simulink model "Ball_and_Plate_MicroLabBox_student_v2019"  (R2019b)
settings: Solver=ode1  StartTime=0.0  StopTime=Inf  FixedStep=0.001  RelTol=1e-3
PostLoadFcn:
  | , if any(exist('dsrtsu_mdlpostloadfcn', 'file') ~= 0), dsrtsu_mdlpostloadfcn('Execute', bdroot); end,
InitFcn:
  | , if any(exist('rtifpga_mdlclblib', 'file') ~= 0), rtifpga_mdlclblib('Init', bdroot); end,
values from neighbouring files (symbols this model uses):
  A_robust = K_robust.A    [Init_workspace.m]    (also in OptimalControlleerSythesisNew.m = K.A)
  B_robust = K_robust.B    [Init_workspace.m]    (also in OptimalControlleerSythesisNew.m = K.B)
  ball_pos_sat = 0.2    [Init_workspace.m]
  ball_vel_sat = 1    [Init_workspace.m]
  Baw_robust = C_robust' / (C_robust*C_robust' + aw_reg*eye(2))    [OptimalControlleerSythesisNew.m]
  C_robust = K_robust.C    [Init_workspace.m]    (also in OptimalControlleerSythesisNew.m = K.C)
  D_robust = K_robust.D    [Init_workspace.m]    (also in OptimalControlleerSythesisNew.m = K.D)
  g = 9.81    [Init_workspace.m]    (also in OptimalControlleerSythesis.m; OptimalControlleerSythesisNew.m; Robustcontroller_angleOutput_Hinf_positionSensitive_center034.m; compute_mpc_params.m)
  K_lqr = dlqr(Ad, Bd, Q_lqr, R_lqr)    [Init_workspace.m]
  Kaw_robust = 0.15    [OptimalControlleerSythesisNew.m]
  path = quintic(-0.0289,3,0,1/fs)    [Init_workspace.m]    (also in Quintic_Time.m = reference_end; Quintic_Velocity.m = reference_end)
  plate_angle_sat = deg2rad(10)    [Init_workspace.m]
  Q_kf = diag([1, 100, 1, 100])    [Init_workspace.m]
  R_kf = diag([0.1, 0.1])    [Init_workspace.m]
  Ts_Outer = 1/50    (= 0.02)    [Init_workspace.m]
  u_max_robust = [ alpha_lim;  beta_lim]    [OptimalControlleerSythesisNew.m]
  u_min_robust = [-alpha_lim; -beta_lim]    [OptimalControlleerSythesisNew.m]
  uA = repmat(uA,[1,P])    [Init_workspace.m]
  uB = repmat(uB,[1,P])    [Init_workspace.m]
  uC = repmat(uC,[1,P])    [Init_workspace.m]
undefined symbols (not defined in the file or in its folder): a_circ, a_square, DiscIntNeverNeededParam, inner_I_sat, r_circ, r_square, Ts_Inner
libraries: simulink x7, rtiemclib x6, rtiethernetlib x3, rti1202lib_dac_class1 x3, slrealtimeutilitieslib x1, mpclib x1
(part 1 of 3)
Description:
  | Standard RTI1202 template.
  | Supported MATLAB version:  R2019b.
settings Model: Tag=RTI1202  DSRTSU_INTERNAL_RTI_VER=570  DSRTSU_INTERNAL_RTI_TYPE=rti1202  RTICANMMDATA=struct('GeneralSetupData',struct('modelroot','C:\git\SystemsAndControlIntegrationProject_5SC25\Experiment\BallANDPlate','generalsettings',struct('filesettings',struct('destfolder',struct('Name','RTICANMM_FILES','Check',1),'buildfolder',struct('Name','.','Check',1),'AbsDestfolder',struct('Name','C:\git\SystemsAndControlIntegrationProject_5SC25\Experiment\BallANDPlate\RTICANMM_FILES'),'AbsBuildfolder',struct('Name','C:\git\SystemsAndControlIntegrationProject_5SC25\Experiment\BallANDPlate'))),'options',struct('addpaths',1,'rmpaths',1,'addtrcexclusion',true,'cannavigator',struct('checkmonitoring',0),'show_usrtrc',0,'use_usrtrc',0),'advanced',struct('options',ones(1,100)),'MPSetup',{{}},'RTI',struct('Type','RTI1202','Ver','7.15','Date','02-Nov-2020'),'modelname','Ball_and_Plate_MicroLabBox_student','block','Ball_and_Plate_MicroLabBox_student'))  DSRTSU_INTERNAL_RTIFPGA=170  Creator=20201603  LastModifiedBy=alexi
settings DataIOCC: ReturnWorkspaceOutputs=off
settings OptimizationCC: BlockReduction=off  OptimizeBlockIOStorage=off  BufferReuse=off  GlobalBufferReuse=off  ExpressionFolding=off  LocalBlockOutputs=off  OptimizeDataStoreBuffers=off  BusAssignmentInplaceUpdate=off
settings DebuggingCC: PregeneratedLibrarySubsystemCodeDiagnostic=none  ArithmeticOperatorsInVariantConditions=warning
settings HardwareCC: ProdBitPerPointer=32  ProdBitPerSizeT=32  ProdBitPerPtrDiffT=32  ProdLargestAtomicInteger=Integer  ProdEndianess=BigEndian  ProdWordSize=32  ProdLongLongMode=on  ProdHWDeviceType=Custom Processor->Custom  TargetIntDivRoundTo=Zero  TargetEndianess=BigEndian  TargetHWDeviceType=Custom Processor->Custom
settings ModelReferenceCC: EnableParallelModelReferenceBuilds=on  ParallelModelReferenceMATLABWorkerInit=Load Top Model
settings SFSimCC: SimUseLocalCustomCode=off  MATLABDynamicMemAlloc=off  CustomCodeUndefinedFunction=UseInterfaceOnly
settings RTWCC: SystemTargetFile=rti1202.tlc  MakeCommand=make_rti  TemplateMakefile=rti1202.tmf  Description=dSPACE DS1202 Hardware Platform  RTWUseLocalCustomCode=off
settings CodeAppCC: StateflowObjectComments=on
settings STFCustomTargetCC: ParMdlRefBuildCompliant=on  SystemTargetFile=rti1202.tlc
settings GRTTargetCC: TargetLangStandard=C89/C90 (ANSI)  CompOptLevelCompliant=off  ConcurrentExecutionCompliant=off  CombineOutputUpdateFcns=off  MatFileLogging=off  CPPClassGenCompliant=off  UseToolchainInfoCompliant=off
settings ConfigComp: CovMetricSettings=dswe  CovBoundaryAbsTol=1.0e-5

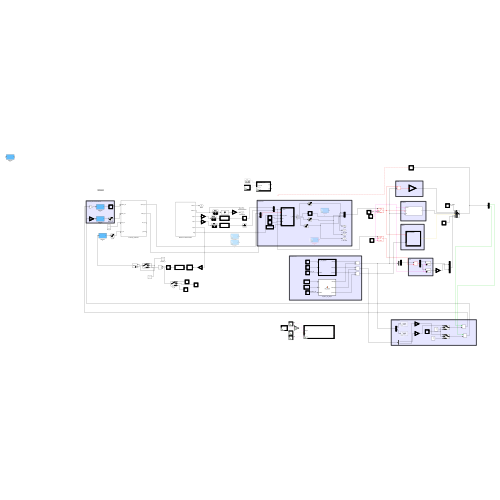
[thumbnail: Simulink's stored preview of the top-level diagram]
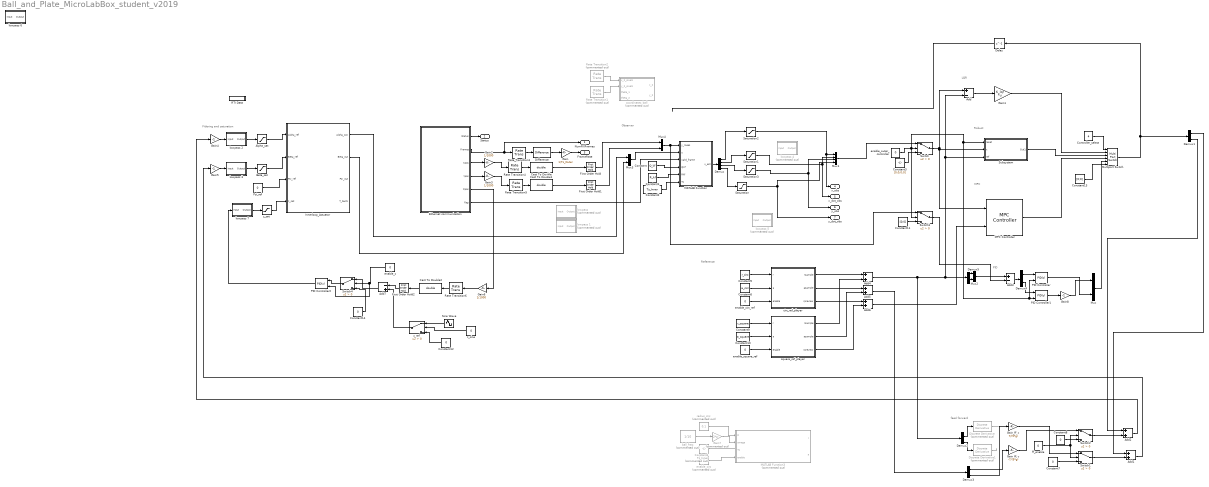
== system Ball_and_Plate_MicroLabBox_student_v2019 ==
  note: PID
  note: MPC
  note: Robust
  note: LQR
  note: feed forward
  note: Reference
  note: Observer
  note: Fitlering and saturation
  Add : Sum  Inputs=+-
  Add{1..2,4..6} (5 alike) : Sum
  Add3 : Sum  Inputs=+-
  Add7 : Sum  Inputs=-+
  "Alpha_sat " : Saturate  UpperLimit=plate_angle_sat  LowerLimit=-plate_angle_sat
  "Beta_sat " : Saturate  UpperLimit=plate_angle_sat  LowerLimit=-plate_angle_sat
  Cast To Double : DataTypeConversion  OutDataTypeStr=double
  Cast To Double1 : DataTypeConversion  OutDataTypeStr=double
  Cast To Double2 : DataTypeConversion  OutDataTypeStr=double
  Constant : Constant  Value=Q_kf
  Constant1 : Constant  Value=R_kf
  Constant10 : Constant  Value=a_square
  Constant11 : Constant  Value=[0;0]
  Constant{7..8,12,14} (4 alike) : Constant  Value=0
  Constant13 : Constant  Value=[0;0]
  Constant2 : Constant  Value=Ts_Inner
  Constant3 : Constant  Value=[0;0;0;0]
  Constant4 : Constant  Commented=on  Value=Ts_Inner
  Constant5 : Constant  Value=r_circ
  Constant6 : Constant  Value=a_circ
  Constant9 : Constant  Value=r_square
  Controller_select : Constant  Value=4
  Delay : Delay  DelayLength=1
  Demux : Demux
  Demux1 : Demux  Outputs=2
  Demux2 : Demux
  Demux3 : Demux  Outputs=2
  Demux4 : Demux  Outputs=2
  Demux5 : Demux
  Difference : simulink/Discrete/Difference  ICPrevInput=0  OutMin=[]  OutMax=[]  OutDataType=fixdt(1, 16)  OutScaling=2^-10  DoSatur=off
  Discrete Derivative : simulink/Discrete/Discrete Derivative  Commented=on  gainval=1.0  ICPrevScaledInput=0.0  OutMin=[]  OutMax=[]  OutDataType=fixdt(1, 16)  OutScaling=2^-10  DoSatur=off
  Discrete Derivative1 : simulink/Discrete/Discrete Derivative  Commented=on  gainval=1.0  ICPrevScaledInput=0.0  OutMin=[]  OutMax=[]  OutDataType=fixdt(1, 16)  OutScaling=2^-10  DoSatur=off
  Ethernet communication : Subsystem
  First Order Hold : FirstOrderHold  ErrorTolerance=inf
  First Order Hold1 : FirstOrderHold  ErrorTolerance=inf
  First Order Hold2 : FirstOrderHold  ErrorTolerance=inf
  Gain : Gain  Gain=1/Ts_Outer
  Gain1 : Gain  Gain=K_lqr  Multiplication=Matrix(K*u)
  Gain2 : Gain  Gain=1/1000
  Gain3 : Gain  Gain=1/1000
  Gain4 : Gain  Gain=-1
  Gain5 : Gain  Gain=-1
  Gain6 : Gain  Gain=1/1000
  Gain7 : Gain  Commented=on  Gain=2*pi
  Gain8 : Gain  Gain=-1
  Gain_ff_x : Gain  Gain=7/(5*g)
  "Gain_ff_y " : Gain  Gain=-7/(5*g)
  Innerloop_Actuator : Subsystem
  MATLAB Function : MATLAB Function  TreatAsAtomicUnit=on
  MATLAB Function3 : MATLAB Function  Commented=on  TreatAsAtomicUnit=on
  MPC Controller : mpclib/MPC Controller  SCDEnableBlockLinearizationSpecification=on  mpcobj=mpcobj  is_multiple=0  enable_value=0  return_u0=off  updateMPCinCallerWorkspace=on  md_inport=off  mv_inport=off  uref_inport=off  return_cost=off  return_mvseq=off  return_qpstatus=off  return_xseq=off  return_state=off  return_ovseq=off  state_inport=on  umin_inport=off  umax_inport=off  ymin_inport=off  ymax_inport=off  cc_inport=off  ywt_inport=off  uwt_inport=off  duwt_inport=off  rhoeps_inport=off  pm_inport=off  MaximumP=10  HorizonChoice=FixedHorizon  n_ts=0.02  n_p=25  n_mv=2  n_md=0  n_ud=0  n_mo=4  n_uo=0  BlockDataType=double  SampleTimeInherited=off  switch_inport=off
  Multiport Switch : MultiPortSwitch  Inputs=5
  Mux{,2..4} (4 alike) : Mux  Inputs=2
  Mux1 : Mux
  PID Controller : simulink/Continuous/PID Controller  Controller=PID  Form=Parallel  TimeDomain=Discrete-time  SampleTime=-1  IntegratorMethod=Forward Euler  FilterMethod=Forward Euler  ControllerParametersSource=internal  P=0.6  I=0.08  D=0.15  N=25  UseFilter=on  TunerSelectOption=Transfer Function Based (PID Tuner App)  InitialConditionSource=internal  InitialConditionForIntegrator=0  InitialConditionForFilter=0  DifferentiatorICPrevScaledInput=0  ExternalReset=rising  TrackingMode=off  Kt=1  LimitOutput=off  UpperSaturationLimit=inf  LowerSaturationLimit=-inf  LinearizeAsGain=on  AntiWindupMode=none  Kb=1  POutMin=[]  POutMax=[]  IOutMin=[]  IOutMax=[]  DOutMin=[]  DOutMax=[]  NOutMin=[]  NOutMax=[]  SumOutMin=[]  SumOutMax=[]  SaturationOutMin=[]  SaturationOutMax=[]  PParamMin=[]  PParamMax=[]  IParamMin=[]  IParamMax=[]  DParamMin=[]  DParamMax=[]  NParamMin=[]  NParamMax=[]  KbParamMin=[]  KbParamMax=[]  KtParamMin=[]  KtParamMax=[]  KbOutMin=[]  KbOutMax=[]  KtOutMin=[]  KtOutMax=[]  IntegratorOutMin=[]  IntegratorOutMax=[]  FilterOutMin=[]  FilterOutMax=[]  SumI1OutMin=[]  SumI1OutMax=[]  SumI2OutMin=[]  SumI2OutMax=[]  SumI3OutMin=[]  SumI3OutMax=[]  SumI4OutMin=[]  SumI4OutMax=[]  SumDOutMin=[]  SumDOutMax=[]  DifferentiatorOutMin=[]  DifferentiatorOutMax=[]  FilterDiffOutCoefMin=[]  FilterDiffOutCoefMax=[]  ReciprocalOutMin=[]  ReciprocalOutMax=[]  SumDenOutMin=[]  SumDenOutMax=[]  SumNumOutMin=[]  SumNumOutMax=[]  DivideOutMin=[]  DivideOutMax=[]  IntegratorContinuousStateAttributes=''  IntegratorStateMustResolveToSignalObject=off  IntegratorRTWStateStorageClass=Auto  FilterContinuousStateAttributes=''  FilterStateMustResolveToSignalObject=off  FilterRTWStateStorageClass=Auto  ParallelPVariant=InternalParameters  IdealPVariant=Disabled  IVariant=InternalParameters  DVariant=InternalParameters  IntegratorVariant=Discrete  SatVariant=Disabled  AWVariant=Passthrough  PCopyVariant=Disabled  TRVariant=Disabled  FdbkBlocksVariant=Forward  IdealPFdbkVariant=Disabled  SatFdbkVariant=Disabled  DerivativeFilterVariant=ForwardEulerFilter  NVariant=InternalParameters  NCopyVariant=Disabled  FilterICVariant=InternalICsFilter  IntegratorICVariant=InternalICs  ExternalResetVariant=ExternalReset  TRSumVariant=Passthrough  SumFdbkVariant=Disabled  SumVariant=Sum_PID
  PID Controller1 : simulink/Continuous/PID Controller  Controller=PID  Form=Parallel  TimeDomain=Discrete-time  SampleTime=-1  IntegratorMethod=Forward Euler  FilterMethod=Forward Euler  ControllerParametersSource=internal  P=0.6  I=0.08  D=0.15  N=25  UseFilter=on  TunerSelectOption=Transfer Function Based (PID Tuner App)  InitialConditionSource=internal  InitialConditionForIntegrator=0  InitialConditionForFilter=0  DifferentiatorICPrevScaledInput=0  ExternalReset=rising  TrackingMode=off  Kt=1  LimitOutput=off  UpperSaturationLimit=inf  LowerSaturationLimit=-inf  LinearizeAsGain=on  AntiWindupMode=none  Kb=1  POutMin=[]  POutMax=[]  IOutMin=[]  IOutMax=[]  DOutMin=[]  DOutMax=[]  NOutMin=[]  NOutMax=[]  SumOutMin=[]  SumOutMax=[]  SaturationOutMin=[]  SaturationOutMax=[]  PParamMin=[]  PParamMax=[]  IParamMin=[]  IParamMax=[]  DParamMin=[]  DParamMax=[]  NParamMin=[]  NParamMax=[]  KbParamMin=[]  KbParamMax=[]  KtParamMin=[]  KtParamMax=[]  KbOutMin=[]  KbOutMax=[]  KtOutMin=[]  KtOutMax=[]  IntegratorOutMin=[]  IntegratorOutMax=[]  FilterOutMin=[]  FilterOutMax=[]  SumI1OutMin=[]  SumI1OutMax=[]  SumI2OutMin=[]  SumI2OutMax=[]  SumI3OutMin=[]  SumI3OutMax=[]  SumI4OutMin=[]  SumI4OutMax=[]  SumDOutMin=[]  SumDOutMax=[]  DifferentiatorOutMin=[]  DifferentiatorOutMax=[]  FilterDiffOutCoefMin=[]  FilterDiffOutCoefMax=[]  ReciprocalOutMin=[]  ReciprocalOutMax=[]  SumDenOutMin=[]  SumDenOutMax=[]  SumNumOutMin=[]  SumNumOutMax=[]  DivideOutMin=[]  DivideOutMax=[]  IntegratorContinuousStateAttributes=''  IntegratorStateMustResolveToSignalObject=off  IntegratorRTWStateStorageClass=Auto  FilterContinuousStateAttributes=''  FilterStateMustResolveToSignalObject=off  FilterRTWStateStorageClass=Auto  ParallelPVariant=InternalParameters  IdealPVariant=Disabled  IVariant=InternalParameters  DVariant=InternalParameters  IntegratorVariant=Discrete  SatVariant=Disabled  AWVariant=Passthrough  PCopyVariant=Disabled  TRVariant=Disabled  FdbkBlocksVariant=Forward  IdealPFdbkVariant=Disabled  SatFdbkVariant=Disabled  DerivativeFilterVariant=ForwardEulerFilter  NVariant=InternalParameters  NCopyVariant=Disabled  FilterICVariant=InternalICsFilter  IntegratorICVariant=InternalICs  ExternalResetVariant=ExternalReset  TRSumVariant=Passthrough  SumFdbkVariant=Disabled  SumVariant=Sum_PID
  PID Controller2 : simulink/Continuous/PID Controller  Controller=PID  Form=Parallel  TimeDomain=Discrete-time  SampleTime=-1  IntegratorMethod=Forward Euler  FilterMethod=Forward Euler  ControllerParametersSource=internal  P=1  I=0  D=0  N=100  UseFilter=on  TunerSelectOption=Transfer Function Based (PID Tuner App)  InitialConditionSource=internal  InitialConditionForIntegrator=0  InitialConditionForFilter=0  DifferentiatorICPrevScaledInput=0  ExternalReset=rising  TrackingMode=off  Kt=1  LimitOutput=off  UpperSaturationLimit=inf  LowerSaturationLimit=-inf  LinearizeAsGain=on  AntiWindupMode=none  Kb=1  POutMin=[]  POutMax=[]  IOutMin=[]  IOutMax=[]  DOutMin=[]  DOutMax=[]  NOutMin=[]  NOutMax=[]  SumOutMin=[]  SumOutMax=[]  SaturationOutMin=[]  SaturationOutMax=[]  PParamMin=[]  PParamMax=[]  IParamMin=[]  IParamMax=[]  DParamMin=[]  DParamMax=[]  NParamMin=[]  NParamMax=[]  KbParamMin=[]  KbParamMax=[]  KtParamMin=[]  KtParamMax=[]  KbOutMin=[]  KbOutMax=[]  KtOutMin=[]  KtOutMax=[]  IntegratorOutMin=[]  IntegratorOutMax=[]  FilterOutMin=[]  FilterOutMax=[]  SumI1OutMin=[]  SumI1OutMax=[]  SumI2OutMin=[]  SumI2OutMax=[]  SumI3OutMin=[]  SumI3OutMax=[]  SumI4OutMin=[]  SumI4OutMax=[]  SumDOutMin=[]  SumDOutMax=[]  DifferentiatorOutMin=[]  DifferentiatorOutMax=[]  FilterDiffOutCoefMin=[]  FilterDiffOutCoefMax=[]  ReciprocalOutMin=[]  ReciprocalOutMax=[]  SumDenOutMin=[]  SumDenOutMax=[]  SumNumOutMin=[]  SumNumOutMax=[]  DivideOutMin=[]  DivideOutMax=[]  IntegratorContinuousStateAttributes=''  IntegratorStateMustResolveToSignalObject=off  IntegratorRTWStateStorageClass=Auto  FilterContinuousStateAttributes=''  FilterStateMustResolveToSignalObject=off  FilterRTWStateStorageClass=Auto  ParallelPVariant=InternalParameters  IdealPVariant=Disabled  IVariant=InternalParameters  DVariant=InternalParameters  IntegratorVariant=Discrete  SatVariant=Disabled  AWVariant=Passthrough  PCopyVariant=Disabled  TRVariant=Disabled  FdbkBlocksVariant=Forward  IdealPFdbkVariant=Disabled  SatFdbkVariant=Disabled  DerivativeFilterVariant=ForwardEulerFilter  NVariant=InternalParameters  NCopyVariant=Disabled  FilterICVariant=InternalICsFilter  IntegratorICVariant=InternalICs  ExternalResetVariant=ExternalReset  TRSumVariant=Passthrough  SumFdbkVariant=Disabled  SumVariant=Sum_PID
  "Psi_ref " : Constant  Value=0
  RTI Data : Subsystem  Tag=struct('RTIDataServer',struct('RTIDataServerVs','2','RTIModelDescription','struct(''main'',''Ball_and_Plate_MicroLabBox_student'',''sub'','''',''isMp'',0)'))  LoadFcn="if exist('rtidc'), try,  rtidc('DataHostBlockClbLoad', gcbh); catch, disp(['Warning: ''LoadFcn'' for RTI Data block failed: ' lasterr]); end, end,"  mask(RTI_DATA_HOST){}
      mask help:
      | RTI Data Block.
      | This block is used by RTI to store internal model-dependent data.
      | Please keep this block on the root level of the model. Deleting this block will result in data loss.
      |
      | NEVER DELETE OR COPY THIS BLOCK!
      settings: CopyFcn="if exist('rtidc'), try,  rtidc('DataHostBlockClbCopy', gcbh); catch, disp(['Warning: ''CopyFcn'' for RTI Data block failed: ' lasterr]); end, end,"  DeleteFcn="if exist('rtidc'), try,  rtidc('DataHostBlockClbDelete', gcbh); catch, disp(['Warning: ''DeleteFcn'' for RTI Data block failed: ' lasterr]); end, end,"  ModelCloseFcn="if exist('rtidc'), try,  rtidc('DataHostBlockClbModelClose', gcbh); catch, disp(['Warning: ''ModelCloseFcn'' for RTI Data block failed: ' lasterr]); end, end,"  PreSaveFcn="if exist('rtidc'), try,  rtidc('DataHostBlockClbPreSave', gcbh); catch, disp(['Warning: ''PreSaveFcn'' for RTI Data block failed: ' lasterr]); end, end,"  PostSaveFcn="if exist('rtidc'), try,  rtidc('DataHostBlockClbPostSave', gcbh); catch, disp(['Warning: ''PostSaveFcn'' for RTI Data block failed: ' lasterr]); end, end,"  NameChangeFcn="if exist('rtidc'), try,  rtidc('DataHostBlockClbNameChange', gcbh); catch, disp(['Warning: ''NameChangeFcn'' for RTI Data block failed: ' lasterr]); end, end,"
      mask Help:
      | RTI Data Block.
      | This block is used by RTI to store internal model-dependent data.
      | Please keep this block on the root level of the model. Deleting this block will result in data loss.
      | 
      | NEVER DELETE OR COPY THIS BLOCK!
      mask Display:
      | text(0.5, 0.5, 'RTI Data', 'HorizontalAlignment', 'center');
      | plot([1 0]);
  Rate Transition1 : RateTransition  Commented=on  Deterministic=off  OutPortSampleTimeMultiple=Ts_Outer  OutPortSampleTime=Ts_Outer
  Rate Transition2 : RateTransition  Commented=on  Deterministic=off  OutPortSampleTimeMultiple=Ts_Outer  OutPortSampleTime=Ts_Outer
  Rate Transition{3..6} (4 alike) : RateTransition  Deterministic=off  OutPortSampleTimeMultiple=Ts_Outer  OutPortSampleTime=Ts_Outer
  Saturation : Saturate  UpperLimit=ball_vel_sat  LowerLimit=-ball_vel_sat
  Saturation1 : Saturate  UpperLimit=ball_vel_sat  LowerLimit=-ball_vel_sat
  Saturation2 : Saturate  UpperLimit=ball_pos_sat  LowerLimit=-ball_pos_sat
  Saturation3 : Saturate  UpperLimit=ball_pos_sat  LowerLimit=-ball_pos_sat
  Sine Wave : Sin  Amplitude=0.005  Frequency=0.5 *2*pi
  Subsystem : Subsystem
  Switch{,1..4} (5 alike) : Switch  Criteria=u2 > Threshold
  ball_freq : Constant  Commented=on  Value=1/10
  "circ_ref_player " : MATLAB Function  TreatAsAtomicUnit=on
  coordinates_ball : MATLAB Function  Commented=on  TreatAsAtomicUnit=on
  enable_circ : Constant  Commented=on  Value=0
  "enable_circ_ref " : Constant  Value=0
  enable_outer_controller : Constant  Value=0
  "enable_square_ref " : Constant  Value=0
  enable_z : Constant  Value=0
  ff_enable : Constant  Value=0
  "lowpass " : Subsystem  Commented=on
  lowpass 1 : Subsystem  Commented=on
  lowpass 2 : Subsystem
  lowpass 3 : Subsystem
  lowpass 4 : Subsystem  Commented=on
  lowpass 5 : Subsystem  Commented=on
  lowpass 6 : Subsystem
  lowpass 7 : Subsystem
  radius_circ : Constant  Commented=on  Value=0.1
  "square_ref_player " : MATLAB Function  TreatAsAtomicUnit=on
  "z_ref " : Switch  Criteria=u2 > Threshold
  "z_sat " : Saturate  UpperLimit=0.02  LowerLimit=-0.02
  "z_sine " : Constant  Value=0
  NumRXFrames : Outport
  Status : Outport  Port=2
  "FrameRate " : Outport  Port=3
  x_obs : Outport  Port=4
  x_dot_obs : Outport  Port=5
  y_obs : Outport  Port=6
  y_dot_obs : Outport  Port=7
  wires:
  Ethernet communication/2("Frames ") -> NumRXFrames/1, Rate Transition3/1
  Rate Transition3/1 -> Difference/1
  Difference/1 -> Gain/1
  Gain/1 -> "FrameRate "/1
  Ethernet communication/1("Status ") -> Status/1
  Rate Transition2/1 -> coordinates_ball/1(x_2_pixels)
  Rate Transition1/1 -> coordinates_ball/2(y_2_pixels)
  "Psi_ref "/1 -> Innerloop_Actuator/3("Psi_ref ")
  Innerloop_Actuator/1(Alpha_out) -> Mux3/1
  Innerloop_Actuator/2(Beta_out) -> Mux3/2
  Demux/1 -> Saturation2/1
  Demux/4 -> Saturation/1
  Demux/3 -> Saturation3/1
  Demux/2 -> Saturation1/1
  Mux1/1 -> Switch/1
  enable_outer_controller/1 -> Switch3/2, PID Controller/2, PID Controller1/2, Subsystem/1("reset "), Switch/2
  Constant3/1 -> Switch/3
  "Alpha_sat "/1 -> Innerloop_Actuator/1("Alpha_ref ")
  "Beta_sat "/1 -> Innerloop_Actuator/2("Beta_ref ")
  Ethernet communication/3("Xpos ") -> Gain2/1
  Ethernet communication/4("Ypos ") -> Gain3/1
  Rate Transition4/1 -> Cast To Double/1
  Rate Transition5/1 -> Cast To Double1/1
  Mux4/1 -> Switch3/1, MATLAB Function/1(y_meas)
  Ethernet communication/6(flag) -> MATLAB Function/3(valid_frame)
  Constant/1 -> MATLAB Function/4(Qkf)
  Constant1/1 -> MATLAB Function/5(Rkf)
  Constant2/1 -> MATLAB Function/6(Ts)
  Gain4/1 -> lowpass 2/1(Input)
  Gain5/1 -> lowpass 3/1(Input)
  Add2/1 -> Gain4/1
  Add1/1 -> Gain5/1
  Saturation2/1 -> Mux1/1, x_obs/1
  Saturation3/1 -> Mux1/3, y_obs/1
  Switch/1 -> MPC Controller/1, Subsystem/2("x "), Add/1
  MATLAB Function/1(x_est) -> Demux/1
  Constant4/1 -> ?
  radius_circ/1 -> MATLAB Function3/1(R)
  ball_freq/1 -> Gain7/1
  Gain7/1 -> MATLAB Function3/2(omega)
  enable_circ/1 -> MATLAB Function3/4(enable)
  Demux2/2 -> Discrete Derivative/1
  Demux2/4 -> Discrete Derivative1/1
  Discrete Derivative1/1 -> ?
  Discrete Derivative/1 -> ?
  Gain_ff_x/1 -> Switch1/1
  Demux1/1 -> Add1/1
  Demux1/2 -> Add2/1
  Switch1/1 -> Add1/2
  ff_enable/1 -> Switch2/2, Switch1/2
  Switch2/1 -> Add2/2
  Constant7/1 -> Switch1/3
  Constant8/1 -> Switch2/3
  "Gain_ff_y "/1 -> Switch2/1
  Gain2/1 -> Rate Transition4/1
  Gain3/1 -> Rate Transition5/1
  First Order Hold1/1 -> Mux4/2
  First Order Hold/1 -> Mux4/1
  Saturation1/1 -> Mux1/2, x_dot_obs/1
  Saturation/1 -> y_dot_obs/1, Mux1/4
  lowpass 2/1(Output) -> "Alpha_sat "/1
  lowpass 3/1(Output) -> "Beta_sat "/1
  Add4/1 -> Demux2/1, Subsystem/3("ref "), Add/2, Demux5/1
  Delay/1 -> ?
  Add/1 -> Gain1/1
  MPC Controller/1 -> Multiport Switch/4
  Subsystem/1(Out1) -> Multiport Switch/3
  Multiport Switch/1 -> Delay/1, Demux1/1
  Gain1/1 -> Multiport Switch/2
  Controller_select/1 -> Multiport Switch/1
  Add3/1 -> Demux4/1
  Demux4/1 -> PID Controller/1
  Demux4/2 -> PID Controller1/1
  Cast To Double/1 -> First Order Hold/1
  Cast To Double1/1 -> First Order Hold1/1
  PID Controller/1 -> Mux/2
  PID Controller1/1 -> Gain8/1
  Gain8/1 -> Mux/1
  Constant5/1 -> "circ_ref_player "/1(r)
  Constant6/1 -> "circ_ref_player "/2(a)
  "enable_circ_ref "/1 -> "circ_ref_player "/3(enable)
  Add5/1 -> Demux3/1
  Mux3/1 -> MATLAB Function/2(u)
  Add6/1 -> MPC Controller/2
  "enable_square_ref "/1 -> "square_ref_player "/3(enable)
  Constant10/1 -> "square_ref_player "/2(a)
  Constant9/1 -> "square_ref_player "/1(r)
  "circ_ref_player "/1(rsample) -> Add4/1
  "square_ref_player "/1(rsample) -> Add4/2
  "circ_ref_player "/2(asample) -> Add5/1
  "square_ref_player "/2(asample) -> Add5/2
  "circ_ref_player "/3(rpreview) -> Add6/1
  "square_ref_player "/3(rpreview) -> Add6/2
  Demux5/1 -> Mux2/1
  Demux5/3 -> Mux2/2
  Constant11/1 -> Switch3/3
  Mux2/1 -> Add3/1
  Switch3/1 -> Add3/2
  Demux3/1 -> "Gain_ff_y "/1
  Demux3/2 -> Gain_ff_x/1
  Mux/1 -> Multiport Switch/5
  Rate Transition6/1 -> Cast To Double2/1
  Gain6/1 -> Rate Transition6/1
  Ethernet communication/5(Zpos) -> Gain6/1
  Cast To Double2/1 -> First Order Hold2/1
  First Order Hold2/1 -> Add7/1
  Add7/1 -> Switch4/1
  enable_z/1 -> PID Controller2/2, Switch4/2
  "z_ref "/1 -> Add7/2
  Switch4/1 -> PID Controller2/1
  PID Controller2/1 -> lowpass 7/1(Input)
  lowpass 7/1(Output) -> "z_sat "/1
  "z_sat "/1 -> Innerloop_Actuator/4("z_set ")
  Constant13/1 -> Multiport Switch/6
  Constant12/1 -> "z_ref "/3
  Sine Wave/1 -> "z_ref "/1
  "z_sine "/1 -> "z_ref "/2
  Constant14/1 -> Switch4/3

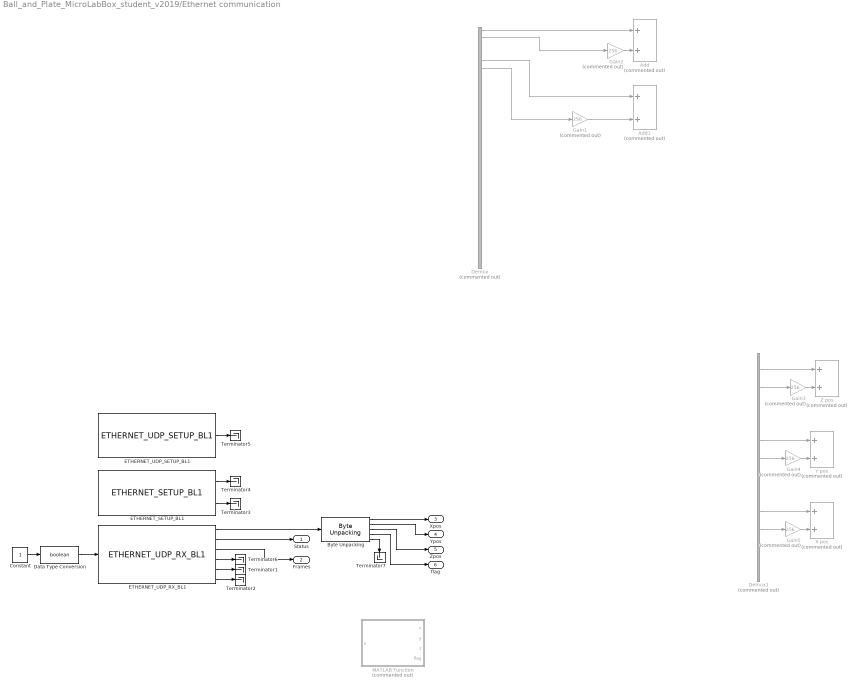
== system Ball_and_Plate_MicroLabBox_student_v2019/Ethernet communication ==
  " X pos" : Sum  Commented=on  AccumDataTypeStr=uint16
  Add : Sum  Commented=on  AccumDataTypeStr=uint16
  Add1 : Sum  Commented=on
  "Byte Unpacking " : slrealtimeutilitieslib/Byte Unpacking  MaskUnpackedDataTypes={'single' 'single' 'single' 'int8' 'int8'}  MaskUnpackedDataSizes={[1],[1],[1],[1],[19]}  MaskAlignment=1
  Constant : Constant
  Data Type Conversion : DataTypeConversion  OutDataTypeStr=boolean
  Demux : Demux  Commented=on  Outputs=32
  Demux1 : Demux  Commented=on  Outputs=12
  ETHERNET_SETUP_BL1 : rtiethernetlib/ETHERNET_SETUP_BL1  DSProperties=struct('RTI',struct('Version',uint32(2),'BlockType',struct('isSLSource',uint8(0),'isSLSink',uint8(0),'isHWSource',uint8(0),'isHWSink',uint8(0),'isSetup',uint8(1),'isInline',uint8(1),'isNonInline',uint8(0),'isInterrupt',uint8(0),'isChannelwise',uint8(0)),'IOBoardType','DSETHERNET','UnitType','ETHERNET','Identifier','SETUP','DialogType','ML','BlockSet','RTIETHERNET','SlaveProcessor','NONE'))  RTIBlockInterface=struct('OutputPortsWidth',int32([3 1 1 4]),'OutputPortsActive',[1 0 0 1],'OutputPortsName',{{['Link Status'],['Watchdog Status'],['DHCP Status'],['Local IP']}},'OutputPortsDataType',{{'SS_UINT32','SS_UINT32','SS_UINT32','SS_UINT8'}},'InitLevel',3,'IconTransparency','on','BlockDisplay',{{['Ethernet Setup\n\nLocal IP: 192.168.140.8'],'left'}},'DialogFcn','rtiethernetsetupgui','BlockName',struct('Token',{{'ETHERNET_SETUP_BL1'}}))  RTIBlockParameters=struct('DHCPserverMode',{{0,'OFF',[0 1]}},'LocalIpNum1',{{'192','OFF',[0 255]}},'LocalIpNum2',{{'168','OFF',[0 255]}},'LocalIpNum3',{{'140','OFF',[0 255]}},'LocalIpNum4',{{'8','OFF',[0 255]}},'SubnetMaskNum1',{{'255','OFF',[0 255]}},'SubnetMaskNum2',{{'255','OFF',[0 255]}},'SubnetMaskNum3',{{'255','OFF',[0 255]}},'SubnetMaskNum4',{{'0','OFF',[0 255]}},'GatewayNum1',{{'0','OFF',[0 255]}},'GatewayNum2',{{'0','OFF',[0 255]}},'GatewayNum3',{{'0','OFF',[0 255]}},'GatewayNum4',{{'0','OFF',[0 255]}},'LinkStatusOutPortMode',{{1,'OFF',[0 1]}},'NumOfEthConnectors',{{3,'ON',[1 16]}},'WatchdogStatusOutPortMode',{{0,'OFF',[0 1]}},'LocalIpOutPortMode',{{1,'OFF',[0 1]}},'IpAndSubmaskCheck',{{int32(1),'OFF',[0 1]}},'TLCFileName',{{'rtiethernetsetup','OFF',[]}})  RTISFcnParameters=struct('DHCPserverMode','int32','LocalIpNum1','uint8','LocalIpNum2','uint8','LocalIpNum3','uint8','LocalIpNum4','uint8','SubnetMaskNum1','uint8','SubnetMaskNum2','uint8','SubnetMaskNum3','uint8','SubnetMaskNum4','uint8','GatewayNum1','uint8','GatewayNum2','uint8','GatewayNum3','uint8','GatewayNum4','uint8','LinkStatusOutPortMode','int32','NumOfEthConnectors','int32','WatchdogStatusOutPortMode','int32','LocalIpOutPortMode','int32','TLCFileName','char')  RTIBlockParaDefault=struct('DHCPserverMode',0,'LocalIpNum1',192,'LocalIpNum2',168,'LocalIpNum3',140,'LocalIpNum4',6,'SubnetMaskNum1',255,'SubnetMaskNum2',255,'SubnetMaskNum3',255,'SubnetMaskNum4',0,'GatewayNum1',0,'GatewayNum2',0,'GatewayNum3',0,'GatewayNum4',0,'LinkStatusOutPortMode',1,'NumOfEthConnectors',3,'WatchdogStatusOutPortMode',0,'LocalIpOutPortMode',0,'IpAndSubmaskCheck',1,'TLCFileName','rtiethernetsetup')
      settings: SourceProductName=dSPACE RTI Ethernet Blockset
  ETHERNET_UDP_RX_BL1 : rtiethernetlib/ETHERNET_UDP_RX_BL1  DSProperties=struct('RTI',struct('Version',uint32(1),'BlockType',struct('isSLSource',uint8(1),'isSLSink',uint8(1),'isHWSource',uint8(0),'isHWSink',uint8(1),'isSetup',uint8(0),'isInline',uint8(1),'isNonInline',uint8(0),'isInterrupt',uint8(0),'isChannelwise',uint8(0)),'IOBoardType','DSETHERNET','UnitType','UDP','Identifier','RXUDP','DialogType','ML','BlockSet','RTIETHERNET','SlaveProcessor','NONE'))  RTIBlockInterface=struct('OutputPortsWidth',int32([32 1 1 1 4 1]),'OutputPortsActive',[1 1 1 1 1 1],'OutputPortsName',{{'Data','Status',['Received Frames'],['Received Bytes'],['Remote IP'],['Remote Port']}},'OutputPortsDataType',{{'SS_UINT8','SS_UINT32','SS_DOUBLE','SS_UINT32','SS_UINT8','SS_UINT16'}},'InputPortsWidth',int32(1),'InputPortsActive',1,'InputPortsName',{{'Enable'}},'InputPortsDataType',{{'SS_BOOLEAN'}},'RWork',{{{'RECEIVED_FRAMES',uint32(1)}}},'InitLevel',3,'IconTransparency','on','BlockDisplay',{{['Ethernet UDP/IP\nRX\n\nSocket ID: 1'],'center'}},'DialogFcn','rtiethernetrxudpgui','BlockName',struct('Token',{{'ETHERNET_UDP_RX_BL1'}}))  RTIBlockParameters=struct('SocketIdIndex',{{2,'OFF',[1 2]}},'SocketId',{{1,'OFF',[-1 inf]}},'RemoteIp',{{['<NOT AVAILABLE>'],'OFF',[]}},'RemotePort',{{['<NOT AVAILABLE>'],'OFF',[]}},'LocalPort',{{49001,'OFF',[]}},'FrameSize',{{'32','OFF',[1 65507]}},'EnableVariableFrameSize',{{1,'OFF',[0 1]}},'VariableFrameSizeMode',{{1,'OFF',[1 2]}},'InterruptMode',{{0,'OFF',[0 1]}},'RemoteIpOutPortMode',{{1,'OFF',[0 1]}},'RemotePortOutPortMode',{{1,'OFF',[0 1]}},'TLCFileName',{{'rtiethernetrxudp','OFF',[]}})  RTISFcnParameters=struct('SocketIdIndex','int32','SocketId','double','FrameSize','uint16','EnableVariableFrameSize','int32','VariableFrameSizeMode','int32','InterruptMode','int32','RemoteIpOutPortMode','int32','RemotePortOutPortMode','int32','TLCFileName','char')  RTIBlockParaDefault=struct('SocketIdIndex',1,'SocketId',-1,'RemoteIp',['<NOT AVAILABLE>'],'RemotePort',['<NOT AVAILABLE>'],'LocalPort',['<NOT AVAILABLE>'],'FrameSize',1024,'EnableVariableFrameSize',0,'VariableFrameSizeMode',1,'InterruptMode',0,'RemoteIpOutPortMode',0,'RemotePortOutPortMode',0,'TLCFileName','rtiethernetrxudp')
      settings: SourceProductName=dSPACE RTI Ethernet Blockset
  ETHERNET_UDP_SETUP_BL1 : rtiethernetlib/ETHERNET_UDP_SETUP_BL1  DSProperties=struct('RTI',struct('Version',uint32(2),'BlockType',struct('isSLSource',uint8(1),'isSLSink',uint8(1),'isHWSource',uint8(0),'isHWSink',uint8(0),'isSetup',uint8(0),'isInline',uint8(1),'isNonInline',uint8(0),'isInterrupt',uint8(0),'isChannelwise',uint8(0)),'IOBoardType','DSETHERNET','UnitType','UDP','Identifier','SETUPUDP','DialogType','ML','BlockSet','RTIETHERNET','SlaveProcessor','NONE'))  RTIBlockInterface=struct('OutputPortsWidth',int32(2),'OutputPortsActive',1,'OutputPortsName',{{['RX Dropped Frames']}},'OutputPortsDataType',{{'SS_DOUBLE'}},'InputPortsWidth',int32([4 1]),'InputPortsActive',int32([0 0]),'InputPortsName',{{['RX Remote IP Filter'],['RX Remote Port Filter']}},'InputPortsDataType',{{'SS_UINT8','SS_UINT16'}},'RWork',{{{'RX_DROPPED_FRAMES',uint32(2)}}},'InitLevel',3,'IconTransparency','on','BlockDisplay',{{['Ethernet UDP/IP\nSetup\n\nSocket ID: 1'],'center'}},'DialogFcn','rtiethernetsetupudpgui','BlockName',struct('Token',{{'ETHERNET_UDP_SETUP_BL1'}}))  RTIBlockParameters=struct('SocketId',{{1,'OFF',[]}},'EnableSocketBind',{{1,'OFF',[0 1]}},'AcceptAnyRxRemoteIp',{{1,'OFF',[0 1]}},'RxRemoteIpNum1',{{'192','OFF',[0 255]}},'RxRemoteIpNum2',{{'168','OFF',[0 255]}},'RxRemoteIpNum3',{{'140','OFF',[0 255]}},'RxRemoteIpNum4',{{'100','OFF',[0 255]}},'EnableDynamicRxRemoteIpFilter',{{0,'OFF',[0 1]}},'AcceptAnyRxRemotePort',{{1,'OFF',[0 1]}},'RxRemotePort',{{'57272','OFF',[1 65535]}},'EnableDynamicRxRemotePortFilter',{{0,'OFF',[0 1]}},'TxRemoteIpNum1',{{'192','OFF',[0 255]}},'TxRemoteIpNum2',{{'168','OFF',[0 255]}},'TxRemoteIpNum3',{{'140','OFF',[0 255]}},'TxRemoteIpNum4',{{'100','OFF',[0 255]}},'TxRemotePort',{{'49002','OFF',[1 65535]}},'SpecifyLocalPort',{{1,'OFF',[0 1]}},'LocalPort',{{'49001','OFF',[1 65535]}},'InterruptMode',{{0,'OFF',[0 1]}},'RxDroppedFramesOutPortMode',{{1,'OFF',[0 1]}},'RemoteIpNumCheck',{{0,'OFF',[0 1]}},'RemotePortCheck',{{0,'OFF',[0 1]}},'LocalPortCheck',{{1,'OFF',[0 1]}},'DHCPserverModeEnabled',{{0,'OFF',[0 1]}},'TLCFileName',{{'rtiethernetsetupudp','OFF',[]}})  RTISFcnParameters=struct('SocketId','double','EnableSocketBind','int32','AcceptAnyRxRemoteIp','int32','RxRemoteIpNum1','uint8','RxRemoteIpNum2','uint8','RxRemoteIpNum3','uint8','RxRemoteIpNum4','uint8','EnableDynamicRxRemoteIpFilter','int32','AcceptAnyRxRemotePort','int32','RxRemotePort','uint16','EnableDynamicRxRemotePortFilter','int32','TxRemoteIpNum1','uint8','TxRemoteIpNum2','uint8','TxRemoteIpNum3','uint8','TxRemoteIpNum4','uint8','TxRemotePort','uint16','SpecifyLocalPort','int32','LocalPort','uint16','InterruptMode','int32','RxDroppedFramesOutPortMode','int32','DHCPserverModeEnabled','int32','TLCFileName','char')  RTIBlockParaDefault=struct('SocketId',-1,'EnableSocketBind',1,'AcceptAnyRxRemoteIp',1,'RxRemoteIpNum1',0,'RxRemoteIpNum2',0,'RxRemoteIpNum3',0,'RxRemoteIpNum4',0,'EnableDynamicRxRemoteIpFilter',0,'AcceptAnyRxRemotePort',1,'RxRemotePort',49002,'EnableDynamicRxRemotePortFilter',0,'TxRemoteIpNum1',0,'TxRemoteIpNum2',0,'TxRemoteIpNum3',0,'TxRemoteIpNum4',0,'TxRemotePort',49002,'SpecifyLocalPort',0,'LocalPort',49001,'InterruptMode',0,'RxDroppedFramesOutPortMode',0,'RemoteIpNumCheck',0,'RemotePortCheck',0,'LocalPortCheck',0,'DHCPserverModeEnabled',0,'TLCFileName','rtiethernetsetupudp')
      settings: SourceProductName=dSPACE RTI Ethernet Blockset
  Gain{1..5} (5 alike) : Gain  Commented=on  Gain=256  OutDataTypeStr=uint16
  MATLAB Function : MATLAB Function  Commented=on  TreatAsAtomicUnit=on
  Terminator{1..7} (7 alike) : Terminator
  Y pos : Sum  Commented=on  AccumDataTypeStr=uint16
  Z pos : Sum  Commented=on  AccumDataTypeStr=uint16
  "Status " : Outport
  "Frames " : Outport  Port=2
  "Xpos " : Outport  Port=3
  "Ypos " : Outport  Port=4
  Zpos : Outport  Port=5
  flag : Outport  Port=6
  wires:
  Demux/1 -> Add/1
  Data Type Conversion/1 -> ETHERNET_UDP_RX_BL1/1
  Demux/2 -> Gain2/1
  Gain1/1 -> Add1/2
  Demux/5 -> Add1/1
  Demux/6 -> Gain1/1
  ETHERNET_UDP_RX_BL1/3 -> "Frames "/1
  Constant/1 -> Data Type Conversion/1
  Gain2/1 -> Add/2
  ETHERNET_UDP_RX_BL1/2 -> "Status "/1
  ETHERNET_SETUP_BL1/1 -> Terminator4/1
  ETHERNET_UDP_RX_BL1/5 -> Terminator1/1
  ETHERNET_UDP_RX_BL1/6 -> Terminator2/1
  ETHERNET_SETUP_BL1/2 -> Terminator3/1
  ETHERNET_UDP_SETUP_BL1/1 -> Terminator5/1
  Gain3/1 -> Z pos/2
  Demux1/1 -> Z pos/1
  Demux1/2 -> Gain3/1
  Gain4/1 -> Y pos/2
  Demux1/5 -> Y pos/1
  Demux1/6 -> Gain4/1
  Gain5/1 -> " X pos"/2
  Demux1/9 -> " X pos"/1
  Demux1/10 -> Gain5/1
  "Byte Unpacking "/2 -> "Ypos "/1
  "Byte Unpacking "/1 -> "Xpos "/1
  "Byte Unpacking "/3 -> Zpos/1
  "Byte Unpacking "/4 -> flag/1
  ETHERNET_UDP_RX_BL1/4 -> Terminator6/1
  ETHERNET_UDP_RX_BL1/1 -> "Byte Unpacking "/1
  "Byte Unpacking "/5 -> Terminator7/1

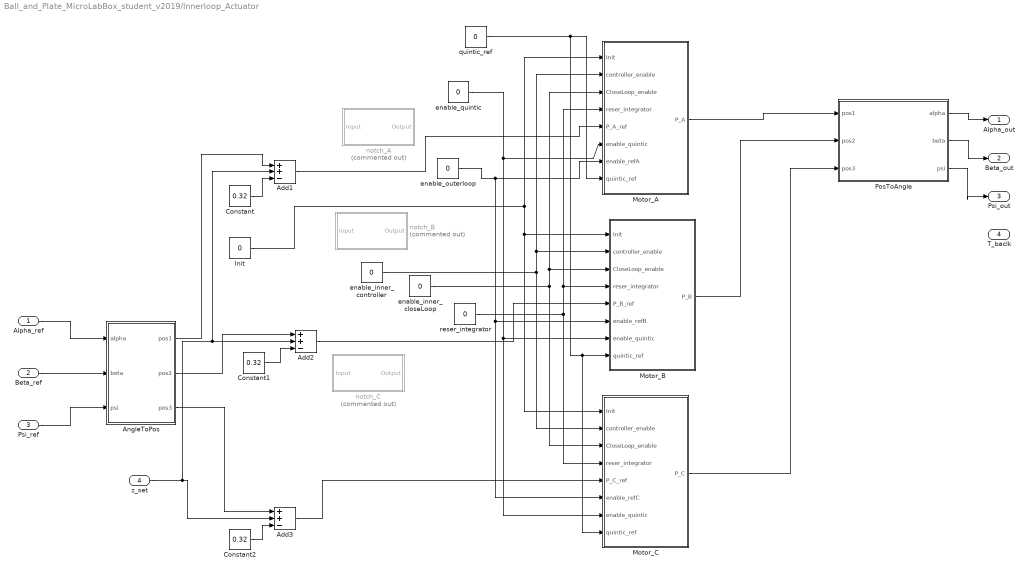
== system Ball_and_Plate_MicroLabBox_student_v2019/Innerloop_Actuator ==
  "Alpha_ref " : Inport
  "Beta_ref " : Inport  Port=2
  "Psi_ref " : Inport  Port=3
  "z_set " : Inport  Port=4
  Add1 : Sum  Inputs=++-
  Add2 : Sum  Inputs=++-
  Add3 : Sum  Inputs=++-
  "AngleToPos " : MATLAB Function  TreatAsAtomicUnit=on
  Constant : Constant  Value=0.32
  Constant1 : Constant  Value=0.32
  Constant2 : Constant  Value=0.32
  "Init " : Constant  Value=0
  Motor_A : Subsystem
  Motor_B : Subsystem
  Motor_C : Subsystem
  "PosToAngle " : MATLAB Function  TreatAsAtomicUnit=on
  enable_inner_closeLoop : Constant  Value=0
  enable_inner_controller : Constant  Value=0
  "enable_outerloop " : Constant  Value=0
  "enable_quintic " : Constant  Value=0
  notch_A : Subsystem  Commented=on
  notch_B : Subsystem  Commented=on
  notch_C : Subsystem  Commented=on
  "quintic_ref " : Constant  Value=0
  reser_integrator : Constant  Value=0
  Alpha_out : Outport
  Beta_out : Outport  Port=2
  Psi_out : Outport  Port=3
  T_baclk : Outport  Port=4
  wires:
  Motor_C/1(P_C) -> "PosToAngle "/3(pos3)
  enable_inner_closeLoop/1 -> Motor_A/3(CloseLoop_enable), Motor_B/3(CloseLoop_enable), Motor_C/3(CloseLoop_enable)
  Constant/1 -> Add1/3
  Constant2/1 -> Add3/3
  Constant1/1 -> Add2/3
  enable_inner_controller/1 -> Motor_A/2(controller_enable), Motor_B/2(controller_enable), Motor_C/2(controller_enable)
  Add3/1 -> Motor_C/5(P_C_ref)
  reser_integrator/1 -> Motor_A/4(reser_integrator), Motor_B/4(reser_integrator), Motor_C/4(reser_integrator)
  Motor_B/1(P_B) -> "PosToAngle "/2(pos2)
  "AngleToPos "/1(pos1) -> Add1/1
  "Alpha_ref "/1 -> "AngleToPos "/1(alpha)
  "Beta_ref "/1 -> "AngleToPos "/2(beta)
  "Psi_ref "/1 -> "AngleToPos "/3(psi)
  "AngleToPos "/2(pos2) -> Add2/1
  "AngleToPos "/3(pos3) -> Add3/1
  "enable_quintic "/1 -> Motor_B/7("enable_quintic "), Motor_C/7("enable_quintic "), Motor_A/6("enable_quintic ")
  "enable_outerloop "/1 -> Motor_C/6(enable_refC), Motor_B/6("enable_refB "), Motor_A/7("enable_refA ")
  "quintic_ref "/1 -> Motor_A/8(quintic_ref), Motor_C/8(quintic_ref), Motor_B/8(quintic_ref)
  "PosToAngle "/3(psi) -> Psi_out/1
  "PosToAngle "/2(beta) -> Beta_out/1
  "PosToAngle "/1(alpha) -> Alpha_out/1
  Motor_A/1(P_A) -> "PosToAngle "/1(pos1)
  Add1/1 -> Motor_A/5("P_A_ref ")
  "Init "/1 -> Motor_B/1(Init), Motor_C/1(Init), Motor_A/1(Init)
  Add2/1 -> Motor_B/5(P_B_ref)
  "z_set "/1 -> Add1/2, Add2/2, Add3/2

== system Ball_and_Plate_MicroLabBox_student_v2019/RTI Data ==
  RTI Data Store : Subsystem  Tag="struct('public',struct('sub',struct('name',{{'Ball_and_Plate_MicroLabBox_student'}},'data',{{struct('TH',struct('thTaskInfo',struct('taskType',{'TIMER','HWINT','TMRINT','SWINT','GLINT'},'tasksNumOf',{1,0,0,0,0},'srcIds',{{'TIMERA'},{},{},{},{}},'taskNames',{{['Timer Task 1']},{},{},{},{}})),'th_tc',struct('dataType','TASK','taskGroupId','','taskGroupList',{{}},'taskSchedulingPolicy','FCFS','taskType','TIMER','blkh',-1,'srcId','TIMERA','srcSgnName',['Timer A interrupt'],'srcCpuName','','taskName',['Timer Task 1  [0.001] s'],'taskNameDisplayExt','','smplTime',0.001,'smplTimeOffs',0,'hasFixedPriority',0,'priority',1,'hasFixedOvc',0,'ovcType',1,'ovcMax',1),'tc_th',struct('dataType','TASK','taskGroupId','','taskGroupList',{{}},'taskSchedulingPolicy','FCFS','taskType','TIMER','blkh',-1,'srcId','TIMERA','srcSgnName',['Timer A interrupt'],'srcCpuName','','taskName',['Timer Task 1  [0.001] s'],'taskNameDisplayExt','','smplTime',0.001,'smplTimeOffs',0,'hasFixedPriority',0,'priority',1,'hasFixedOvc',0,'ovcType',1,'ovcMax',1))}})),'private',struct('version',struct('dsVer',uint32(2)),'access',struct('modified',['26-Jun-2026 14:41:37'],'type','Model','isPerm',1)))"  mask(RTI_DATA_STORE){}
      mask help:
      | RTI Data Store Block. This block is used by RTI to store internal model dependent data. Deleting this block will result in data loss.
      |
      | NEVER DELETE, COPY, OR MODIFY THIS BLOCK!
      mask Help:
      | RTI Data Store Block. This block is used by RTI to store internal model dependent data. Deleting this block will result in data loss.
      | 
      | NEVER DELETE, COPY, OR MODIFY THIS BLOCK!
      mask Display: text(0.5, 0.5, ' ', 'HorizontalAlignment', 'center');

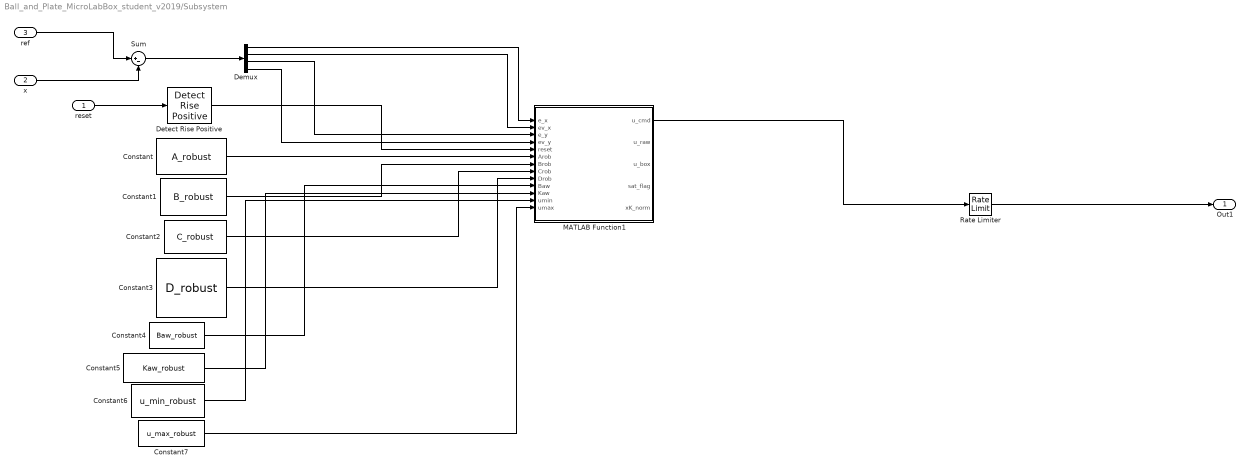
== system Ball_and_Plate_MicroLabBox_student_v2019/Subsystem ==
  "reset " : Inport
  "x " : Inport  Port=2
  "ref " : Inport  Port=3
  Constant : Constant  Value=A_robust  SampleTime=Ts_Outer
  Constant1 : Constant  Value=B_robust  SampleTime=Ts_Outer
  Constant2 : Constant  Value=C_robust  SampleTime=Ts_Outer
  Constant3 : Constant  Value=D_robust  SampleTime=Ts_Outer
  Constant4 : Constant  Value=Baw_robust  SampleTime=Ts_Outer
  Constant5 : Constant  Value=Kaw_robust  SampleTime=Ts_Outer
  Constant6 : Constant  Value=u_min_robust  SampleTime=Ts_Outer
  Constant7 : Constant  Value=u_max_robust  SampleTime=Ts_Outer
  Demux : Demux
  Detect Rise Positive : simulink/Logic and Bit Operations/Detect Rise Positive  vinit=0  OutDataTypeStr=boolean
  MATLAB Function1 : MATLAB Function  TreatAsAtomicUnit=on
  Rate Limiter : RateLimiter  RisingSlewLimit=deg2rad(12)  FallingSlewLimit=-deg2rad(12)  SampleTimeMode=inherited
  Sum : Sum  Inputs=|+-
  Out1 : Outport
  wires:
  Constant/1 -> MATLAB Function1/6(Arob)
  Constant1/1 -> MATLAB Function1/7(Brob)
  Constant2/1 -> MATLAB Function1/8(Crob)
  Constant3/1 -> MATLAB Function1/9(Drob)
  Constant4/1 -> MATLAB Function1/10(Baw)
  Constant5/1 -> MATLAB Function1/11(Kaw)
  Constant6/1 -> MATLAB Function1/12(umin)
  Constant7/1 -> MATLAB Function1/13(umax)
  Detect Rise Positive/1 -> MATLAB Function1/5(reset)
  "reset "/1 -> Detect Rise Positive/1
  Demux/1 -> MATLAB Function1/1(e_x)
  Demux/2 -> MATLAB Function1/2(ev_x)
  Demux/3 -> MATLAB Function1/3(e_y)
  Demux/4 -> MATLAB Function1/4(ev_y)
  "ref "/1 -> Sum/1
  "x "/1 -> Sum/2
  Sum/1 -> Demux/1
  MATLAB Function1/1(u_cmd) -> Rate Limiter/1
  Rate Limiter/1 -> Out1/1

== system Ball_and_Plate_MicroLabBox_student_v2019/lowpass  ==
  Input : Inport
  Dct1lowpass2 : S-Function  FunctionName=dlowpass1  Parameters=f_den, 0.001  SFunctionDeploymentMode=off  EnableBusSupport=off  mask(dctools){f_den=30}
      mask prompts: f_den "Pole [Hz]"
      mask help: This block implements a discrete time 1st order lowpass filter.
      mask Display: disp('DCT 1st order lowpass')
  Gain1 : Gain  SaturateOnIntegerOverflow=on  OutDataTypeStr=Inherit: Same as input  ParamDataTypeStr=Inherit: Same as input
  Output : Outport
  wires:
  Input/1 -> Gain1/1
  Gain1/1 -> Dct1lowpass2/1
  Dct1lowpass2/1 -> Output/1

== system Ball_and_Plate_MicroLabBox_student_v2019/lowpass 1 ==
  Input : Inport
  Dct1lowpass2 : S-Function  FunctionName=dlowpass1  Parameters=f_den, 0.001  SFunctionDeploymentMode=off  EnableBusSupport=off  mask(dctools){f_den=30}
      mask prompts: f_den "Pole [Hz]"
      mask help: This block implements a discrete time 1st order lowpass filter.
      mask Display: disp('DCT 1st order lowpass')
  Gain1 : Gain  SaturateOnIntegerOverflow=on  OutDataTypeStr=Inherit: Same as input  ParamDataTypeStr=Inherit: Same as input
  Output : Outport
  wires:
  Input/1 -> Gain1/1
  Gain1/1 -> Dct1lowpass2/1
  Dct1lowpass2/1 -> Output/1

== system Ball_and_Plate_MicroLabBox_student_v2019/lowpass 2 ==
  Input : Inport
  Dct1lowpass2 : S-Function  FunctionName=dlowpass1  Parameters=f_den, 0.001  SFunctionDeploymentMode=off  EnableBusSupport=off  mask(dctools){f_den=1/Ts_Outer}
      mask prompts: f_den "Pole [Hz]"
      mask help: This block implements a discrete time 1st order lowpass filter.
      mask Display: disp('DCT 1st order lowpass')
  Gain1 : Gain  SaturateOnIntegerOverflow=on  OutDataTypeStr=Inherit: Same as input  ParamDataTypeStr=Inherit: Same as input
  Output : Outport
  wires:
  Input/1 -> Gain1/1
  Gain1/1 -> Dct1lowpass2/1
  Dct1lowpass2/1 -> Output/1

== system Ball_and_Plate_MicroLabBox_student_v2019/lowpass 3 ==
  Input : Inport
  Dct1lowpass2 : S-Function  FunctionName=dlowpass1  Parameters=f_den, 0.001  SFunctionDeploymentMode=off  EnableBusSupport=off  mask(dctools){f_den=1/Ts_Outer}
      mask prompts: f_den "Pole [Hz]"
      mask help: This block implements a discrete time 1st order lowpass filter.
      mask Display: disp('DCT 1st order lowpass')
  Gain1 : Gain  SaturateOnIntegerOverflow=on  OutDataTypeStr=Inherit: Same as input  ParamDataTypeStr=Inherit: Same as input
  Output : Outport
  wires:
  Input/1 -> Gain1/1
  Gain1/1 -> Dct1lowpass2/1
  Dct1lowpass2/1 -> Output/1

== system Ball_and_Plate_MicroLabBox_student_v2019/lowpass 4 ==
  Input : Inport
  Dct1lowpass2 : S-Function  FunctionName=dlowpass1  Parameters=f_den, 0.001  SFunctionDeploymentMode=off  EnableBusSupport=off  mask(dctools){f_den=50}
      mask prompts: f_den "Pole [Hz]"
      mask help: This block implements a discrete time 1st order lowpass filter.
      mask Display: disp('DCT 1st order lowpass')
  Gain1 : Gain  SaturateOnIntegerOverflow=on  OutDataTypeStr=Inherit: Same as input  ParamDataTypeStr=Inherit: Same as input
  Output : Outport
  wires:
  Input/1 -> Gain1/1
  Gain1/1 -> Dct1lowpass2/1
  Dct1lowpass2/1 -> Output/1

== system Ball_and_Plate_MicroLabBox_student_v2019/lowpass 5 ==
  Input : Inport
  Dct1lowpass2 : S-Function  FunctionName=dlowpass1  Parameters=f_den, 0.001  SFunctionDeploymentMode=off  EnableBusSupport=off  mask(dctools){f_den=50}
      mask prompts: f_den "Pole [Hz]"
      mask help: This block implements a discrete time 1st order lowpass filter.
      mask Display: disp('DCT 1st order lowpass')
  Gain1 : Gain  SaturateOnIntegerOverflow=on  OutDataTypeStr=Inherit: Same as input  ParamDataTypeStr=Inherit: Same as input
  Output : Outport
  wires:
  Input/1 -> Gain1/1
  Gain1/1 -> Dct1lowpass2/1
  Dct1lowpass2/1 -> Output/1

== system Ball_and_Plate_MicroLabBox_student_v2019/lowpass 6 ==
  Input : Inport
  Dct1lowpass2 : S-Function  FunctionName=dlowpass1  Parameters=f_den, 0.001  SFunctionDeploymentMode=off  EnableBusSupport=off  mask(dctools){f_den=25}
      mask prompts: f_den "Pole [Hz]"
      mask help: This block implements a discrete time 1st order lowpass filter.
      mask Display: disp('DCT 1st order lowpass')
  Gain1 : Gain  SaturateOnIntegerOverflow=on  OutDataTypeStr=Inherit: Same as input  ParamDataTypeStr=Inherit: Same as input
  Output : Outport
  wires:
  Input/1 -> Gain1/1
  Gain1/1 -> Dct1lowpass2/1
  Dct1lowpass2/1 -> Output/1

== system Ball_and_Plate_MicroLabBox_student_v2019/lowpass 7 ==
  Input : Inport
  Dct1lowpass2 : S-Function  FunctionName=dlowpass1  Parameters=f_den, 0.001  SFunctionDeploymentMode=off  EnableBusSupport=off  mask(dctools){f_den=1}
      mask prompts: f_den "Pole [Hz]"
      mask help: This block implements a discrete time 1st order lowpass filter.
      mask Display: disp('DCT 1st order lowpass')
  Gain1 : Gain  SaturateOnIntegerOverflow=on  OutDataTypeStr=Inherit: Same as input  ParamDataTypeStr=Inherit: Same as input
  Output : Outport
  wires:
  Input/1 -> Gain1/1
  Gain1/1 -> Dct1lowpass2/1
  Dct1lowpass2/1 -> Output/1

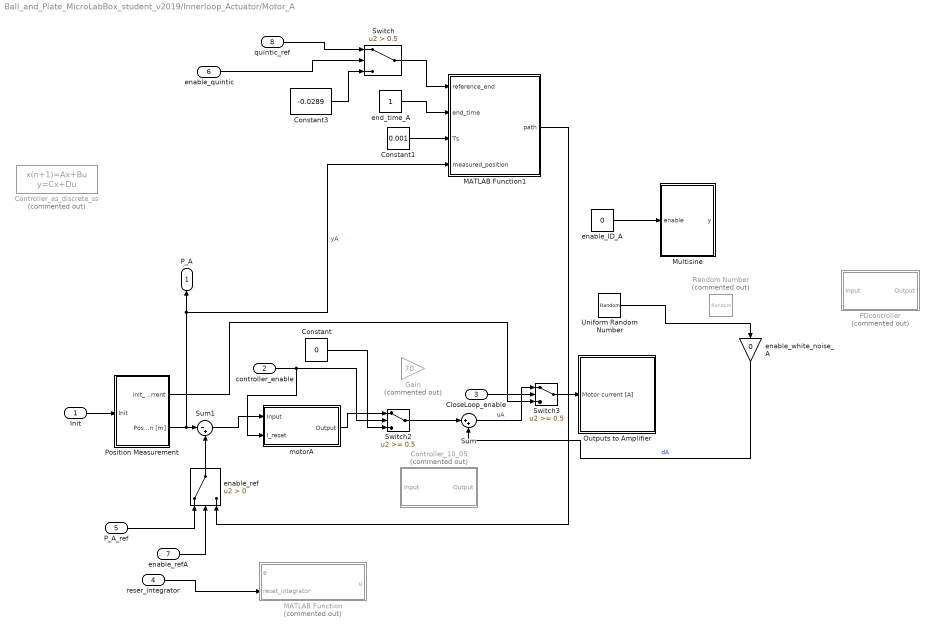
== system Ball_and_Plate_MicroLabBox_student_v2019/Innerloop_Actuator/Motor_A ==
  Init : Inport
  controller_enable : Inport  Port=2
  CloseLoop_enable : Inport  Port=3
  reser_integrator : Inport  Port=4
  "P_A_ref " : Inport  Port=5
  "enable_quintic " : Inport  Port=6
  "enable_refA " : Inport  Port=7
  quintic_ref : Inport  Port=8
  Constant : Constant  Value=0
  Constant1 : Constant  Value=0.001
  Constant3 : Constant  Value=-0.0289
  Controller_10_05 : Subsystem  Commented=on
  Controller_as_discrete_ss : DiscreteStateSpace  Commented=on  A=[0.5498,0.8818;0,0.8543]  B=[5.1803;10.8938]  C=[-5.1480,10.8259]  D=63.6008  SampleTime=-1
  Gain : Gain  Commented=on  Gain=70
  MATLAB Function : MATLAB Function  Commented=on  TreatAsAtomicUnit=on
  MATLAB Function1 : MATLAB Function  TreatAsAtomicUnit=on
  Multisine : Subsystem
  Outputs to Amplifier : Subsystem  TreatAsAtomicUnit=on
  PDcontroller : Subsystem  Commented=on
  Position Measurement : Subsystem  TreatAsAtomicUnit=on
  Random Number : RandomNumber  Commented=on  Variance=0.5
  Sum : Sum  Inputs=|++
  Sum1 : Sum  Inputs=|-+  SaturateOnIntegerOverflow=on
  Switch : Switch  Criteria=u2 > Threshold  Threshold=0.5
  Switch2 : Switch  Threshold=0.5
  Switch3 : Switch  Threshold=0.5
  Uniform Random Number : UniformRandomNumber  Minimum=-2.4  Maximum=2.4
  "enable_ID_A " : Constant  Value=0
  "enable_ref " : Switch  Criteria=u2 > Threshold
  "enable_white_noise_A " : Gain  Gain=0
  end_time_A : Constant
  "motorA " : Subsystem
  P_A : Outport
  wires:
  "motorA "/1(Output) -> Switch2/1
  Switch3/1 -> Outputs to Amplifier/1(Motor current [A])
  Position Measurement/2(Position [m]) -> MATLAB Function1/4(measured_position), P_A/1, Sum1/1  "yA"
  Position Measurement/1(init_current) -> Switch3/3
  CloseLoop_enable/1 -> Switch3/2
  reser_integrator/1 -> MATLAB Function/2(reset_integrator)
  Sum1/1 -> "motorA "/1(Input)
  Constant/1 -> Switch2/3
  controller_enable/1 -> "motorA "/2(I_reset), Switch2/2
  "P_A_ref "/1 -> "enable_ref "/1
  Init/1 -> Position Measurement/1(Init)
  "enable_ID_A "/1 -> Multisine/1(enable)
  Switch2/1 -> Sum/1
  Sum/1 -> Switch3/1  "uA"
  Uniform Random Number/1 -> "enable_white_noise_A "/1
  "enable_ref "/1 -> Sum1/2
  "enable_refA "/1 -> "enable_ref "/2
  Constant1/1 -> MATLAB Function1/3(Ts)
  end_time_A/1 -> MATLAB Function1/2(end_time)
  Constant3/1 -> Switch/3
  Switch/1 -> MATLAB Function1/1(reference_end)
  quintic_ref/1 -> Switch/1
  "enable_quintic "/1 -> Switch/2
  MATLAB Function1/1(path) -> "enable_ref "/3
  "enable_white_noise_A "/1 -> Sum/2  "dA"

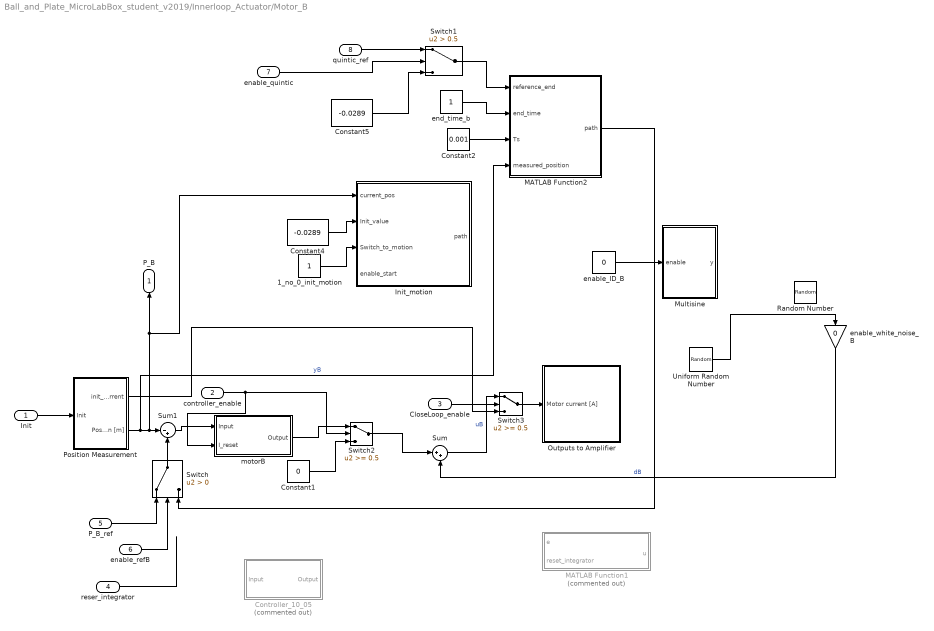
== system Ball_and_Plate_MicroLabBox_student_v2019/Innerloop_Actuator/Motor_B ==
  Init : Inport
  controller_enable : Inport  Port=2
  CloseLoop_enable : Inport  Port=3
  reser_integrator : Inport  Port=4
  P_B_ref : Inport  Port=5
  "enable_refB " : Inport  Port=6
  "enable_quintic " : Inport  Port=7
  quintic_ref : Inport  Port=8
  1_no_0_init_motion : Constant
  Constant1 : Constant  Value=0
  Constant2 : Constant  Value=0.001
  Constant4 : Constant  Value=-0.0289
  Constant5 : Constant  Value=-0.0289
  Controller_10_05 : Subsystem  Commented=on
  Init_motion : Subsystem
  MATLAB Function1 : MATLAB Function  Commented=on  TreatAsAtomicUnit=on
  MATLAB Function2 : MATLAB Function  TreatAsAtomicUnit=on
  Multisine : Subsystem
  Outputs to Amplifier : Subsystem  TreatAsAtomicUnit=on
  Position Measurement : Subsystem  TreatAsAtomicUnit=on
  Random Number : RandomNumber  Variance=0.5
  Sum : Sum  Inputs=|++
  Sum1 : Sum  Inputs=|-+  SaturateOnIntegerOverflow=on
  Switch : Switch  Criteria=u2 > Threshold
  Switch1 : Switch  Criteria=u2 > Threshold  Threshold=0.5
  Switch2 : Switch  Threshold=0.5
  Switch3 : Switch  Threshold=0.5
  Uniform Random Number : UniformRandomNumber  Minimum=-1.8  Maximum=1.8
  "enable_ID_B " : Constant  Value=0
  "enable_white_noise_B " : Gain  Gain=0
  "end_time_b " : Constant
  motorB : Subsystem
  P_B : Outport
  wires:
  motorB/1(Output) -> Switch2/1
  Switch3/1 -> Outputs to Amplifier/1(Motor current [A])
  Position Measurement/2(Position [m]) -> MATLAB Function2/4(measured_position), Init_motion/1(current_pos), P_B/1, Sum1/1  "yB"
  Position Measurement/1(init_current) -> Switch3/3
  Switch2/1 -> Sum/1
  CloseLoop_enable/1 -> Switch3/2
  Sum1/1 -> motorB/1(Input)
  controller_enable/1 -> motorB/2(I_reset), Switch2/2
  Constant1/1 -> Switch2/3
  Init/1 -> Position Measurement/1(Init)
  reser_integrator/1 -> ?
  "enable_ID_B "/1 -> Multisine/1(enable)
  Sum/1 -> Switch3/1  "uB"
  "enable_white_noise_B "/1 -> Sum/2  "dB"
  Constant4/1 -> Init_motion/2(Init_value)
  1_no_0_init_motion/1 -> Init_motion/3(Switch_to_motion)
  Switch/1 -> Sum1/2
  P_B_ref/1 -> Switch/1
  "enable_refB "/1 -> Switch/2
  "end_time_b "/1 -> MATLAB Function2/2(end_time)
  Switch1/1 -> MATLAB Function2/1(reference_end)
  Constant2/1 -> MATLAB Function2/3(Ts)
  MATLAB Function2/1(path) -> Switch/3
  quintic_ref/1 -> Switch1/1
  Constant5/1 -> Switch1/3
  "enable_quintic "/1 -> Switch1/2
  Uniform Random Number/1 -> "enable_white_noise_B "/1
